simulink model "sample"  (Simulink 8.3)
settings: Solver=ode45  StartTime=0.0  StopTime=5  MaxStep=0.005  RelTol=1e-3
settings Model: Creator=Administrator  LastModifiedBy=Administrator
settings DataIOCC: SignalLoggingSaveFormat=Dataset
settings DebuggingCC: UnderspecifiedInitializationDetection=Simplified  StateNameClashWarn=none
settings GRTTargetCC: CombineOutputUpdateFcns=on  GRTInterface=off

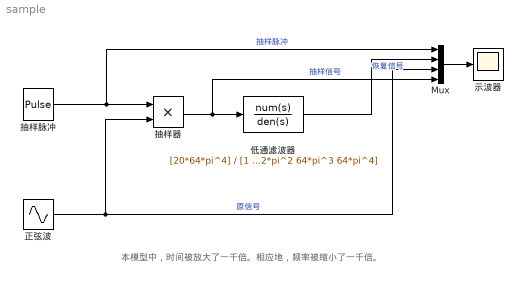
== system sample ==
  note: 本模型中，时间被放大了一千倍。相应地，频率被缩小了一千倍。
  Mux : Mux
  低通滤波器 : TransferFcn  Numerator=[20*64*pi^4]  Denominator=[1 8*pi 32*pi^2 64*pi^3 64*pi^4]
  抽样器 : Product
  抽样脉冲 : DiscretePulseGenerator  PulseType=Time based  Period=0.125  PulseWidth=10
  正弦波 : Sin  Frequency=pi*4  Phase=pi/2  SampleTime=0
  示波器 : Scope
      settings: ShowLegends=on  TimeRange=5
  wires:
  抽样脉冲/1 -> Mux/1, 抽样器/1  "抽样脉冲"
  正弦波/1 -> Mux/3, 抽样器/2  "原信号"
  Mux/1 -> 示波器/1
  抽样器/1 -> Mux/4, 低通滤波器/1  "抽样信号"
  低通滤波器/1 -> Mux/2  "恢复信号"
